simulink model "project"  (R2021a)
settings: Solver=VariableStepAuto  StartTime=0.0  StopTime=10  RelTol=1e-3
values from neighbouring files (symbols this model uses):
  c = Simulink.Parameter(200)    [script.m]
  d = Simulink.Parameter(1)    [script.m]
  H = Simulink.Parameter(3e-2)    [script.m]
  J = Simulink.Parameter(1)    [script.m]
  k = Simulink.Parameter(20)    [script.m]
  Kb = Simulink.Parameter(1)    [script.m]
  Kt = Simulink.Parameter(1)    [script.m]
  L = Simulink.Parameter(1)    [script.m]
  La = Simulink.Parameter(1)    [script.m]
  len = Simulink.Parameter(5e-2)    [script.m]
  m = Simulink.Parameter(40)    [script.m]
  M = Simulink.Parameter(1)    [script.m]
  N = Simulink.Parameter(1)    [script.m]
  R = Simulink.Parameter(1)    [script.m]
  Ra = Simulink.Parameter(1)    [script.m]
  theta = Simulink.Parameter(0)    [script.m]
  v = Simulink.Parameter(3)    [script.m]
settings Model: OrderedModelArguments=off  Creator=adrian  LastModifiedBy=adrian

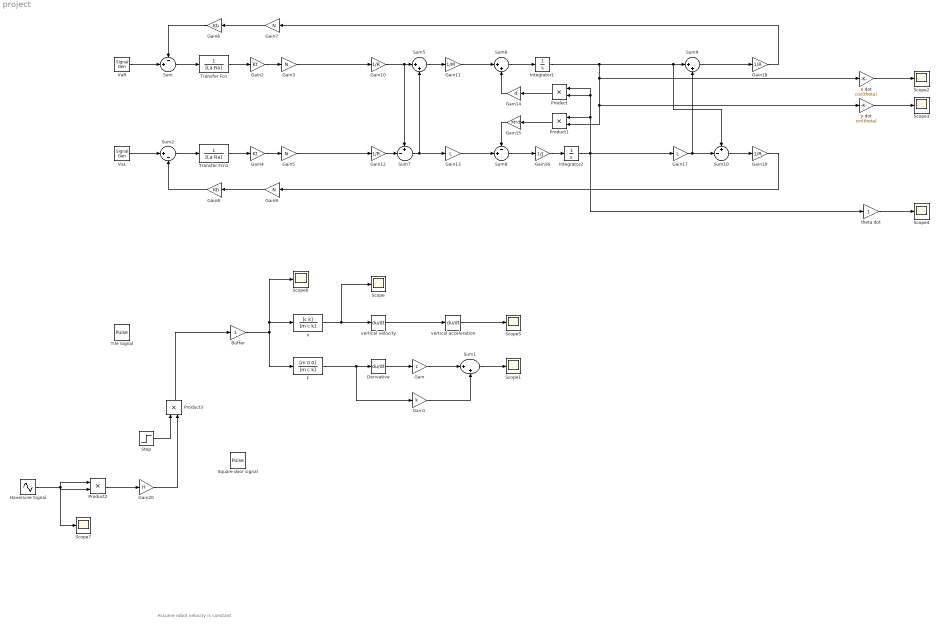
== system project ==
  note: Assume robot velocity is constant
  Buffer : Gain
  Derivative : Derivative
  F : TransferFcn  Numerator=[m 0 0]  Denominator=[m c k]
  Gain : Gain  Gain=c
  Gain1 : Gain  Gain=k
  Gain{10,12,18..19} (4 alike) : Gain  Gain=1/R
  Gain11 : Gain  Gain=1/M
  Gain13 : Gain  Gain=L
  Gain14 : Gain  Gain=d
  Gain15 : Gain  Gain=M*d
  Gain16 : Gain  Gain=1/J
  Gain17 : Gain  Gain=L
  Gain2 : Gain  Gain=Kt
  Gain20 : Gain  Gain=H
  Gain{3,5,7,9} (4 alike) : Gain  Gain=N
  Gain4 : Gain  Gain=Kt
  Gain6 : Gain  Gain=Kb
  Gain8 : Gain  Gain=Kb
  Haversine Signal : Sin  Frequency=pi * v / len  SampleTime=0
  Integrator1 : Integrator
  Integrator2 : Integrator
  Product{,1..3} (4 alike) : Product
  Scope{,1..7} (8 alike) : Scope
  Square door signal : DiscretePulseGenerator  PulseType=Time based  Amplitude=H  Period=(len * 2) / v  PulseWidth=50
  Step : Step  Time=len / v  Before=1  After=0  SampleTime=0
  Sum : Sum  Inputs=-+|
  Sum{1,5..6,9} (4 alike) : Sum  Inputs=|++
  Sum10 : Sum  Inputs=+-|
  Sum2 : Sum  Inputs=|+-
  Sum7 : Sum  Inputs=+-|
  Sum8 : Sum  Inputs=-+|
  Tile Signal : DiscretePulseGenerator  PulseType=Time based  Amplitude=0.005  Period=0.3148 / v  PulseWidth=30.48 / 31.48 * 100
  Transfer Fcn : TransferFcn  Denominator=[La Ra]
  Transfer Fcn1 : TransferFcn  Denominator=[La Ra]
  VaL : SignalGenerator  Units=rad/sec
  VaR : SignalGenerator  Units=rad/sec
  theta dot : Gain
  vertical acceleration : Derivative
  vertical velocity : Derivative
  x : TransferFcn  Numerator=[c k]  Denominator=[m c k]
  x dot : Gain  Gain=cos(theta)
  y dot : Gain  Gain=sin(theta)
  wires:
  VaR/1 -> Sum/2
  Sum/1 -> Transfer Fcn/1
  Transfer Fcn/1 -> Gain2/1
  Gain2/1 -> Gain3/1
  Gain4/1 -> Gain5/1
  Transfer Fcn1/1 -> Gain4/1
  Sum2/1 -> Transfer Fcn1/1
  VaL/1 -> Sum2/1
  Gain7/1 -> Gain6/1
  Gain6/1 -> Sum/1
  Gain9/1 -> Gain8/1
  Gain8/1 -> Sum2/2
  Gain10/1 -> Sum7/1, Sum5/1
  Sum5/1 -> Gain11/1
  Gain11/1 -> Sum6/1
  Sum6/1 -> Integrator1/1
  Sum7/1 -> Gain13/1, Sum5/2
  Sum8/1 -> Gain16/1
  Gain12/1 -> Sum7/2
  Product1/1 -> Gain15/1
  Product/1 -> Gain14/1
  Gain14/1 -> Sum6/2
  Gain13/1 -> Sum8/2
  Gain15/1 -> Sum8/1
  Gain16/1 -> Integrator2/1
  Integrator1/1 -> y dot/1, Product1/2, x dot/1, Sum10/1, Sum9/1
  Integrator2/1 -> theta dot/1, Product1/1, Product/2, Product/1, Gain17/1
  Gain17/1 -> Sum9/2, Sum10/2
  Sum10/1 -> Gain19/1
  Sum9/1 -> Gain18/1
  Gain3/1 -> Gain10/1
  Gain5/1 -> Gain12/1
  Gain19/1 -> Gain9/1
  Gain18/1 -> Gain7/1
  x/1 -> Scope/1, vertical velocity/1
  vertical velocity/1 -> vertical acceleration/1
  F/1 -> Gain1/1, Derivative/1
  Derivative/1 -> Gain/1
  Gain1/1 -> Sum1/2
  Gain/1 -> Sum1/1
  Sum1/1 -> Scope1/1
  theta dot/1 -> Scope4/1
  y dot/1 -> Scope3/1
  x dot/1 -> Scope2/1
  vertical acceleration/1 -> Scope5/1
  Haversine Signal/1 -> Scope7/1, Product2/2, Product2/1
  Product2/1 -> Gain20/1
  Step/1 -> Product3/1
  Buffer/1 -> F/1, x/1, Scope6/1
  Product3/1 -> Buffer/1
  Gain20/1 -> Product3/2
